simulink model "BBB_Accel_Test"  (R2013a)
settings: Solver=FixedStepDiscrete  StartTime=0.0  StopTime=inf  FixedStep=0.01  RelTol=1e-3
settings Model: SimulationMode=external  ExtModeTrigDuration=100  Creator=rdustinkahawita  LastModifiedBy=rdustinkahawita
settings OptimizationCC: OptimizeModelRefInitCode=on  LifeSpan=Inf
settings DebuggingCC: SolverPrmCheckMsg=none  StrictBusMsg=Warning
settings HardwareCC: ProdLargestAtomicInteger=Long  ProdLargestAtomicFloat=Double  ProdEndianess=LittleEndian  ProdHWDeviceType=ARM Compatible->ARM Cortex
settings SFSimCC: SimBuildMode=sf_make_clean
settings RTWCC: SystemTargetFile=realtime.tlc  GenerateMakefile=off  TemplateMakefile=realtime.tmf  Description=Run on Target Hardware  RTWVerbose=off  ProcessScript=realtime_make_rtw_hook
settings STFCustomTargetCC: TargetLibSuffix=.a  GenerateSampleERTMain=on  ERTCustomFileBanners=on  SupportNonInlinedSFcns=off  SupportVariableSizeSignals=on  MATLABClassNameForMDSCustomization=Simulink.SoftwareTarget.ERTCustomization  SystemTargetFile=realtime.tlc
settings ERTTargetCC: ParMdlRefBuildCompliant=off  CompOptLevelCompliant=off  ConcurrentExecutionCompliant=off  CombineOutputUpdateFcns=off  ERTFirstTimeCompliant=off  SupportContinuousTime=on  SupportVariableSizeSignals=on  ModelStepFunctionPrototypeControlCompliant=off  CPPClassGenCompliant=off  ExtMode=on  ExtModeMexArgs='192.168.7.2' 0 17725  ERTSrcFileBannerTemplate=realtime_code_template.cgt  ERTHdrFileBannerTemplate=realtime_code_template.cgt  ERTDataSrcFileTemplate=realtime_code_template.cgt  ERTDataHdrFileTemplate=realtime_code_template.cgt  ERTCustomFileTemplate=realtime_file_process.tlc

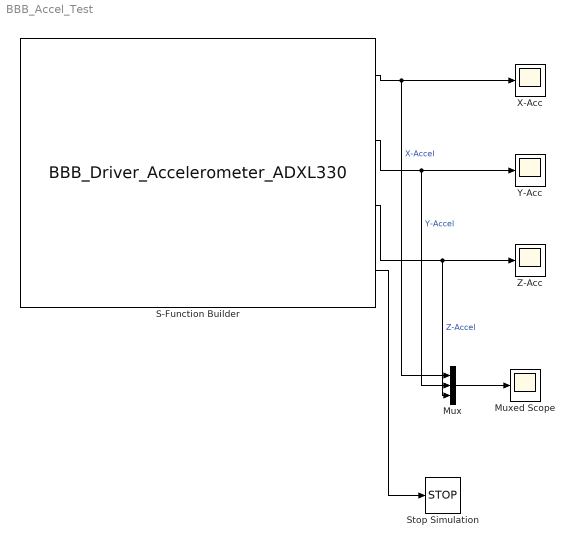
== system BBB_Accel_Test ==
  Mux : Mux  Inputs=3
  Muxed Scope : Scope
      settings: ShowLegends=on  TimeRange=30  YMin=-0.4  YMax=2  SaveName=ScopeData3
  S-Function Builder : S-Function  InitFcn=try, set_param(gcb,'FunctionName','BBB_Driver_Accelerometer_ADXL330'), end  FunctionName=BBB_Driver_Accelerometer_ADXL330  Parameters=uint16(2),boolean(1),uint16(6)  SFunctionModules=BBB_Driver_Accelerometer_ADXL330_wrapper  EnableBusSupport=off  mask(S-Function Builder){}
      mask help: Simulink:masks:SFunctionBuilder_MD
      mask init:
      | val = [[.9  0.75 0.75 1 1 .9 .9 1]',[1 1 0.75 0.75 .9 .9 1 .9]'];try , sys = get_param(gcb,'SfunBuilderFcnName');if isempty(sys), sys = get_param(gcb,'FunctionName'); end,catch, sys = get_param(gcb,'FunctionName'); end
      settings: CopyFcn=set_param(gcbh,'LinkStatus','none')  PreSaveFcn=try, set_param(gcb,'FunctionName','BBB_Driver_Accelerometer_ADXL330'), end  OpenFcn=sfunctionwizard(gcbh)
      mask Display: plot(val(:,1),val(:,2)),disp(sys), port_label('output',1,'outX_Axis_Accel'), port_label('output',2,'outY_Axis_Accel'), port_label('output',3,'outZ_Axis_Accel'), port_label('output',4,'outSimStop')
  Stop Simulation : Stop
  "X-Acc " : Scope
      settings: YMin=-0.2  YMax=0.15
  Y-Acc : Scope
      settings: YMin=-2.75  YMax=0.5
  Z-Acc : Scope
      settings: SaveName=ScopeData2
  wires:
  S-Function Builder/1 -> Mux/1, "X-Acc "/1  "X-Accel"
  S-Function Builder/2 -> Y-Acc/1, Mux/2  "Y-Accel"
  S-Function Builder/3 -> Mux/3, Z-Acc/1  "Z-Accel"
  Mux/1 -> Muxed Scope/1
  S-Function Builder/4 -> Stop Simulation/1
